simulink model "week2_2016741077_ImSeYeong_simul"  (R2021a)
settings: Solver=VariableStepAuto  StartTime=0.0  StopTime=0.1  RelTol=1e-3
values from neighbouring files (symbols this model uses):
  b = J/t    (= 0.00264627659574)    [week2_2016741077_ImSeYeong.m]
  J = 99.5*10^-2*10^-2*10^-3    (= 9.95e-06)    [week2_2016741077_ImSeYeong.m]
  Ke = 68.3*10^-3    (= 0.0683)    [week2_2016741077_ImSeYeong.m]
  Kt = 68.3*10^-3    (= 0.0683)    [week2_2016741077_ImSeYeong.m]
  La = 0.658*10^-3    (= 0.000658)    [week2_2016741077_ImSeYeong.m]
  Ra = 1.76    [week2_2016741077_ImSeYeong.m]
  Tl = 0    [week2_2016741077_ImSeYeong.m]
  Tl05 = 0.5    [week2_2016741077_ImSeYeong.m]
  Tl1 = 1    [week2_2016741077_ImSeYeong.m]
  Va12 = 12    [week2_2016741077_ImSeYeong.m]
  Va24 = 24    [week2_2016741077_ImSeYeong.m]
  Va48 = 48    [week2_2016741077_ImSeYeong.m]
  Va5 = 5    [week2_2016741077_ImSeYeong.m]
settings Model: Creator=syl12  LastModifiedBy=syl12

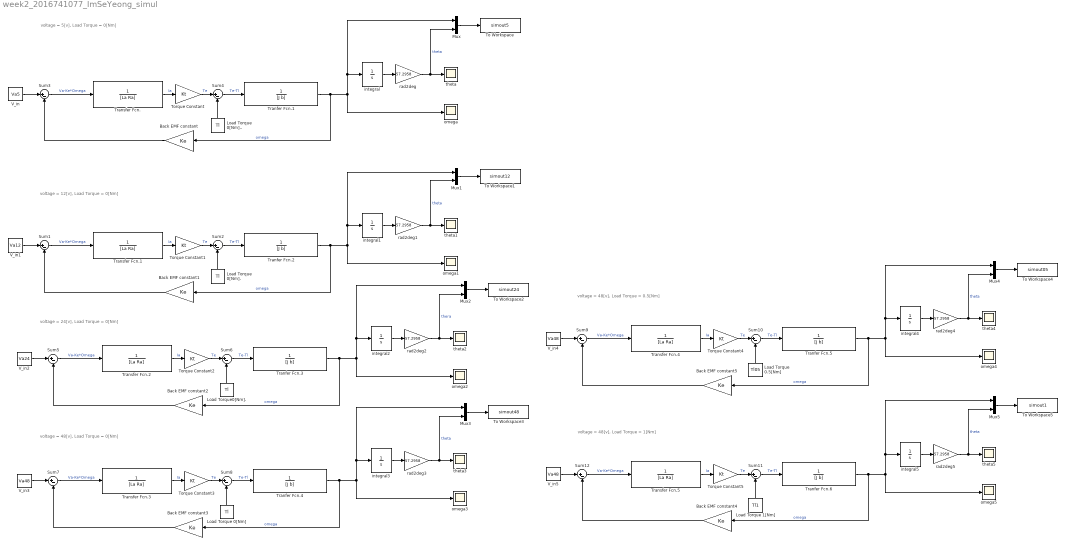
== system week2_2016741077_ImSeYeong_simul ==
  note: voltage = 48[v], Load Torque = 1[Nm]
  note: voltage = 48[v], Load Torque = 0.5[Nm]
  note: voltage = 48[v], Load Torque = 0[Nm]
  note: voltage = 24[v], Load Torque = 0[Nm]
  note: voltage = 12[v], Load Torque = 0[Nm]
  note: voltage = 5[v], Load Torque = 0[Nm]
  Back EMF constant{,1..5} (6 alike) : Gain  Gain=Ke
  Load Torque 0.5[Nm] : Constant  Value=Tl05
  Load Torque 0[Nm] : Constant  Value=Tl
  Load Torque 0[Nm]. : Constant  Value=Tl
  Load Torque 0[Nm].. : Constant  Value=Tl
  Load Torque 1[Nm] : Constant  Value=Tl1
  Load Torque0[Nm]. : Constant  Value=Tl
  Mux{,1..5} (6 alike) : Mux  Inputs=2
  Sum{1..12} (12 alike) : Sum  Inputs=|+-
  To Workspace : ToWorkspace  VariableName=simout5  SaveFormat=Structure With Time  SampleTime=-1
  To Workspace1 : ToWorkspace  VariableName=simout12  SaveFormat=Structure With Time  SampleTime=-1
  To Workspace2 : ToWorkspace  VariableName=simout24  SaveFormat=Structure With Time  SampleTime=-1
  To Workspace3 : ToWorkspace  VariableName=simout48  SaveFormat=Structure With Time  SampleTime=-1
  To Workspace4 : ToWorkspace  VariableName=simout05  SaveFormat=Structure With Time  SampleTime=-1
  To Workspace5 : ToWorkspace  VariableName=simout1  SaveFormat=Structure With Time  SampleTime=-1
  Torque Constant{,1..5} (6 alike) : Gain  Gain=Kt
  Tranfer Fcn.{1..6} (6 alike) : TransferFcn  Denominator=[J b]
  Transfer Fcn.{,1..5} (6 alike) : TransferFcn  Denominator=[La Ra]
  V_in : Constant  Value=Va5
  V_in1 : Constant  Value=Va12
  V_in2 : Constant  Value=Va24
  V_in3 : Constant  Value=Va48
  V_in4 : Constant  Value=Va48
  V_in5 : Constant  Value=Va48
  integral{,1..5} (6 alike) : TransferFcn  Denominator=[1 0]
  omega{,1..5} (6 alike) : Scope
  rad2deg{,1..5} (6 alike) : Gain  Gain=57.2958
  theta{,1..5} (6 alike) : Scope
  wires:
  Tranfer Fcn.1/1 -> integral/1, Mux/1, omega/1, Back EMF constant/1  "omega"
  Sum4/1 -> Tranfer Fcn.1/1  "Te-Tl"
  V_in/1 -> Sum3/1
  Back EMF constant/1 -> Sum3/2
  Load Torque 0[Nm]../1 -> Sum4/2
  Torque Constant/1 -> Sum4/1  "Te"
  Sum3/1 -> Transfer Fcn./1  "Va-Ke*Omega"
  Transfer Fcn./1 -> Torque Constant/1  "Ia"
  Mux/1 -> To Workspace/1
  integral/1 -> rad2deg/1
  rad2deg/1 -> Mux/2, theta/1  "theta"
  Transfer Fcn.1/1 -> Torque Constant1/1  "Ia"
  Tranfer Fcn.2/1 -> integral1/1, Mux1/1, omega1/1, Back EMF constant1/1  "omega"
  Sum1/1 -> Transfer Fcn.1/1  "Va-Ke*Omega"
  integral1/1 -> rad2deg1/1
  Torque Constant1/1 -> Sum2/1  "Te"
  Back EMF constant1/1 -> Sum1/2
  V_in1/1 -> Sum1/1
  Mux1/1 -> To Workspace1/1
  Load Torque 0[Nm]./1 -> Sum2/2
  rad2deg1/1 -> Mux1/2, theta1/1  "theta"
  Sum2/1 -> Tranfer Fcn.2/1  "Te-Tl"
  Transfer Fcn.2/1 -> Torque Constant2/1  "Ia"
  Tranfer Fcn.3/1 -> integral2/1, Mux2/1, omega2/1, Back EMF constant2/1  "omega"
  Sum5/1 -> Transfer Fcn.2/1  "Va-Ke*Omega"
  integral2/1 -> rad2deg2/1
  Torque Constant2/1 -> Sum6/1  "Te"
  Back EMF constant2/1 -> Sum5/2
  V_in2/1 -> Sum5/1
  Mux2/1 -> To Workspace2/1
  Load Torque0[Nm]./1 -> Sum6/2
  rad2deg2/1 -> Mux2/2, theta2/1  "thera"
  Sum6/1 -> Tranfer Fcn.3/1  "Te-Tl"
  Transfer Fcn.3/1 -> Torque Constant3/1  "Ia"
  Tranfer Fcn.4/1 -> integral3/1, Mux3/1, omega3/1, Back EMF constant3/1  "omega"
  Sum7/1 -> Transfer Fcn.3/1  "Va-Ke*Omega"
  integral3/1 -> rad2deg3/1
  Torque Constant3/1 -> Sum8/1  "Te"
  Back EMF constant3/1 -> Sum7/2
  V_in3/1 -> Sum7/1
  Mux3/1 -> To Workspace3/1
  Load Torque 0[Nm]/1 -> Sum8/2
  rad2deg3/1 -> Mux3/2, theta3/1  "theta"
  Sum8/1 -> Tranfer Fcn.4/1  "Te-Tl"
  Sum10/1 -> Tranfer Fcn.5/1  "Te-Tl"
  rad2deg4/1 -> Mux4/2, theta4/1  "theta"
  V_in4/1 -> Sum9/1
  Load Torque 0.5[Nm]/1 -> Sum10/2
  Tranfer Fcn.5/1 -> integral4/1, Mux4/1, omega4/1, Back EMF constant5/1  "omega"
  Mux4/1 -> To Workspace4/1
  Torque Constant4/1 -> Sum10/1  "Te"
  Back EMF constant5/1 -> Sum9/2
  integral4/1 -> rad2deg4/1
  Sum9/1 -> Transfer Fcn.4/1  "Va-Ke*Omega"
  Transfer Fcn.4/1 -> Torque Constant4/1  "Ia"
  integral5/1 -> rad2deg5/1
  Transfer Fcn.5/1 -> Torque Constant5/1  "Ia"
  Sum12/1 -> Transfer Fcn.5/1  "Va-Ke*Omega"
  Back EMF constant4/1 -> Sum12/2
  Torque Constant5/1 -> Sum11/1  "Te"
  V_in5/1 -> Sum12/1
  Tranfer Fcn.6/1 -> integral5/1, Mux5/1, omega5/1, Back EMF constant4/1  "omega"
  Mux5/1 -> To Workspace5/1
  Load Torque 1[Nm]/1 -> Sum11/2
  Sum11/1 -> Tranfer Fcn.6/1  "Te-Tl"
  rad2deg5/1 -> Mux5/2, theta5/1  "theta"
